simulink model "TriggeredEnabled_Subsystem2"  (R2017b)
settings: Solver=FixedStepDiscrete  StartTime=0.0  StopTime=100  FixedStep=1.000000  RelTol=1e-3  EnableMultiTasking=on
model workspace (MAT data in the model file):
  already_pp = 0
  input_struct.time = [0; 1; 2; 3; 4; 5; 6; 7; 8; 9; 10; 11; 12; 13; 14; 15; 16; 17; 18; 19; 20; 21; 22; 23; 24; 25; 26; 27; 28; 29; 30; 31; 32; 33; 34; 35; 36; 37; 38; 39; 40; 41; 42; 43; 44; 45; 46; 47; 48; 49; 50; 51; 52; 53; 54; 55; 56; 57; 58; 59; 60; 61; 62; 63; 64; 65; 66; 67; 68; 69; 70; 71; 72; 73; 74; 75; 76; 77; 78; 79; 80; 81; 82; 83; 84; 85; 86; 87; 88; 89; 90; 91; 92; 93; 94; 95; 96; 97; 98; 99]
  input_struct.signals(1).name = 'In1'
  input_struct.signals(1).values = [3.98063722648; 53.2624225205; -32.7566800611; 25.1970240426; -34.6195984366; -37.7786302223; 29.2156795728; -13.2616735513; -79.4226903861; -52.7698066696; 94.3565591819; 39.779483265; 31.8900511745; -34.7805316897; -96.0356165618; 14.0945183957; -92.7330196105; -47.051451026; -61.8683131624; -10.1400751156; 53.7310357926; 25.5872394796; -37.059941435; -41.5913730898; -84.3524022995; -65.6112333468; 44.2560690434; -82.1102826535; 83.5624405583; -14.064609817; -84.0554257535; 14.4288227563; 66.3544628597; -30.5264390293; 55.9778008647; 41.6678460224; 18.1884717707; -24.6012607537; -21.2349950474; -14.338230833; -15.3948782012; -56.2151433266; -0.647069584082; -92.026057304; 12.9632997433; -90.1714081216; 74.4562486666; 72.0049519433; -32.3484114206; 94.806092687; 90.9550016107; 97.7241995084; -68.456465051; -99.4163299412; -50.3640079277; -30.7419758547; -53.3322574395; 51.1782368274; -54.8144635915; -10.3113509135; -48.1110866803; -30.8410972286; 80.5909895771; -97.4598263468; -73.5554391665; -22.3874691414; 68.1242020715; -57.346739418; 87.0468795352; 93.9600758032; -24.9482888275; 96.9725684633; -75.5828610838; 52.1914940202; 15.8723366272; 24.2313084936; -2.0191519107; -55.9099292253; -71.173151092; 27.0351410609; 60.4831387036; 33.9286517968; -5.67940848208; 88.8956228926; 18.2961735178; -54.6504481273; 36.7687374427; -35.871428846; 49.7837087618; 99.6286414749; -46.0533296631; 86.3739271561; 39.2774105964; -80.9481433314; -50.8255655544; 86.9315103101; -4.04315637288; 76.5055487274; 55.8594633547; -96.343223048]
  input_struct.signals(1).dimensions = 1
  input_struct.signals(2).name = 'Enable'
  input_struct.signals(2).values = [1; 1; 1; 1; 1; 0; 0; 0; 0; 0; 0; 0; 0; 1; 1; 1; 0; 1; 1; 0; 1; 0; 1; 0; 1; 0; 1; 0; 1; 0; 0; 1; 0; 1; 1; 1; 1; 0; 0; 0; 1; 1; 0; 1; 1; 0; 0; 0; 1; 1; 0; 1; 0; 1; 1; 1; 1; 0; 1; 0; 0; 1; 0; 0; 1; 0; 1; 0; 0; 1; 1; 0; 0; 0; 1; 0; 0; 1; 1; 1; 0; 1; 1; 1; 1; 0; 1; 0; 0; 0; 0; 0; 1; 1; 0; 0; 0; 0; 0; 0]
  input_struct.signals(2).dimensions = 1
  input_struct.signals(3).name = 'Trigger'
  input_struct.signals(3).values = [1; 1; 1; 0; 0; 0; 1; 1; 1; 0; 0; 0; 1; 1; 0; 0; 0; 1; 1; 1; 1; 0; 0; 0; 1; 0; 0; 0; 1; 1; 0; 1; 1; 1; 0; 1; 1; 0; 0; 0; 1; 0; 0; 0; 0; 1; 0; 1; 0; 0; 0; 0; 1; 1; 0; 1; 0; 1; 0; 1; 0; 1; 0; 0; 0; 1; 0; 1; 0; 0; 1; 0; 0; 0; 1; 1; 0; 0; 1; 0; 1; 0; 0; 1; 1; 0; 1; 1; 1; 1; 1; 0; 0; 0; 0; 0; 1; 0; 1; 1]
  input_struct.signals(3).dimensions = 1
settings Model: Creator=hbourbou  LastModifiedBy=hbourbou
settings DataIOCC: ExternalInput=input_struct  LoadExternalInput=on  SaveFormat=StructureWithTime
settings OptimizationCC: LifeSpan=inf
settings DebuggingCC: AlgebraicLoopMsg=error  ArtificialAlgebraicLoopMsg=error  SFExecutionAtInitializationDiag=none
settings HardwareCC: ProdBitPerSizeT=32  ProdBitPerPtrDiffT=32  ProdWordSize=32  ProdHWDeviceType=Specified
settings CodeAppCC: StateflowObjectComments=on

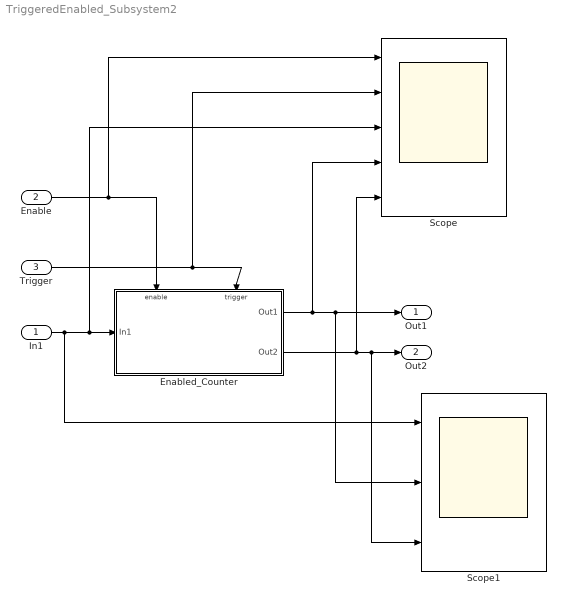
== system TriggeredEnabled_Subsystem2 ==
  In1 : Inport  OutDataTypeStr=double  PortDimensions=1
  Enable : Inport  Port=2  OutDataTypeStr=boolean  PortDimensions=1
  Trigger : Inport  Port=3  OutDataTypeStr=boolean  PortDimensions=1
  Enabled_Counter : Subsystem  TreatAsAtomicUnit=on
  Scope : Scope  NumInputPorts=5
  Scope1 : Scope  NumInputPorts=3
  Out1 : Outport
  Out2 : Outport  Port=2
  wires:
  Enabled_Counter/2(Out2) -> Scope/5, Scope1/3, Out2/1
  Enable/1 -> Scope/1, Enabled_Counter/Enable
  In1/1 -> Scope1/1, Scope/3, Enabled_Counter/1(In1)
  Trigger/1 -> Scope/2, Enabled_Counter/Trigger
  Enabled_Counter/1(Out1) -> Scope/4, Scope1/2, Out1/1

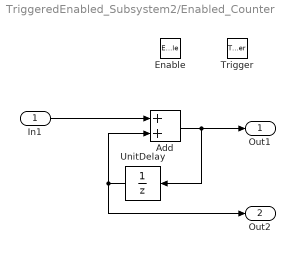
== system TriggeredEnabled_Subsystem2/Enabled_Counter ==
  In1 : Inport  OutDataTypeStr=double  PortDimensions=1
  Enable : EnablePort  StatesWhenEnabling=reset
  Trigger : TriggerPort  VariantControl=(inherit)  PortDimensions=1
  Add : Sum
  UnitDelay : UnitDelay  SampleTime=-1
  Out1 : Outport  InitialOutput=0
  Out2 : Outport  Port=2
  wires:
  UnitDelay/1 -> Out2/1, Add/2
  In1/1 -> Add/1
  Add/1 -> UnitDelay/1, Out1/1
